simulink model "task3"  (R2016a)
settings: Solver=VariableStepAuto  StartTime=0.0  StopTime=10.0  RelTol=1e-3
libraries: dspquant2 x2, dsparch4 x1
settings Model: Creator=Misachu  LastModifiedBy=Misachu

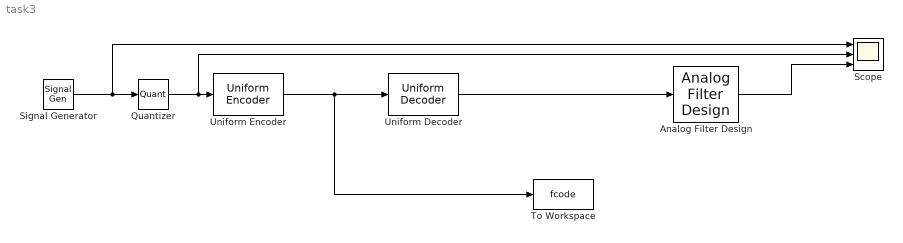
== system task3 ==
  Analog Filter Design : dsparch4/Analog Filter Design  method=Butterworth  filttype=Lowpass  N=8  Wlo=30  Whi=80  Rp=2  Rs=40
  Quantizer : Quantizer
  Scope : Scope  NumInputPorts=3
  Signal Generator : SignalGenerator  Units=rad/sec
  To Workspace : ToWorkspace  VariableName=fcode  SaveFormat=Timeseries  SampleTime=-1
  Uniform Decoder : dspquant2/Uniform Decoder  peak=1  bits=3  overflowMode=Saturate  otype=Double
  Uniform Encoder : dspquant2/Uniform Encoder  peak=1  bits=8  otype=Unsigned integer
  wires:
  Signal Generator/1 -> Scope/1, Quantizer/1
  Quantizer/1 -> Scope/2, Uniform Encoder/1
  Uniform Encoder/1 -> To Workspace/1, Uniform Decoder/1
  Uniform Decoder/1 -> Analog Filter Design/1
  Analog Filter Design/1 -> Scope/3
